simulink model "comunicacionesTarea2"  (R2021a)
settings: Solver=VariableStepAuto  StartTime=0.0  StopTime=0.5  RelTol=1e-3
libraries: spsTriangleGeneratorLib x1
settings Model: Creator=jmata  LastModifiedBy=jmata

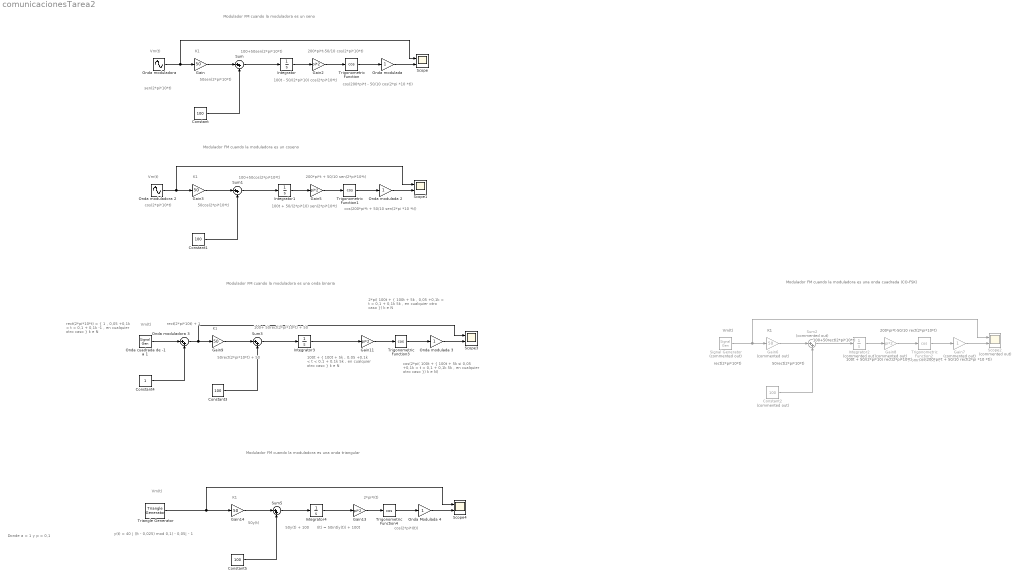
== system comunicacionesTarea2 ==
  note: cos(2*pi*I(t))
  note: 2*pi*I(t)
  note: I(t) = 50int(y(t)) + 100t
  note: 50y(t) + 100
  note: 50y(t)
  note: y(t) = 40 | ((t - 0,025) mod 0,1) - 0,05| - 1
  note: Donde a = 1 y p = 0,1
  note: 2*pi( 100t + {
      |
      | 100t + 5k , 0,05 +0,1k < t < 0,1 + 0,1k
      |
      | 5k , en cualquier otro caso
      |
      | }) k e N
  note: rect(2*pi*10t) + 1
  note: Modulador FM cuando la moduladora es una onda cuadrada (CO-FSK)
  note: Modulador FM cuando la moduladora es un coseno
  note: cos(200*pi*t - 50/10 cos(2*pi *10 *t))
  note: 200*pi*t-50/10 cos(2*pi*10*t)
  note: 100t - 50/(2*pi*10) cos(2*pi*10*t)
  note: 100+50sen(2*pi*10*t)
  note: 50sen(2*pi*10*t)
  note: sen(2*pi*10*t)
  note: Modulador FM cuando la moduladora es un seno
  note: K1
  note: Vm(t)
  note: 50cos(2*pi*10*t)
  note: 100t + 50/(2*pi*10) sen(2*pi*10*t)
  note: 100+50cos(2*pi*10*t)
  note: K1
  note: Vm(t)
  note: cos(200*pi*t + 50/10 sen(2*pi *10 *t))
  note: cos(2*pi*10*t)
  note: 200*pi*t + 50/10 sen(2*pi*10*t)
  note: 100+50rect(2*pi*10*t)
  note: rect(2*pi*10*t)
  note: cos(200*pi*t + 50/10 rect(2*pi *10 *t))
  note: 50rect(2*pi*10*t)
  note: 100t + 50/(2*pi*10) rect(2*pi*10*t)
  note: 200*pi*t-50/10 rect(2*pi*10*t)
  note: K1
  note: Vm(t)
  note: 50rect(2*pi*10*t) + 50
  note: 100+ 50rect(2*pi*10*t) + 50
  note: 100t + {
      |
      | 100t + 5k , 0,05 +0,1k < t < 0,1 + 0,1k
      |
      | 5k , en cualquier otro caso
      |
      | } k e N
  note: K1
  note: cos(2*pi( 100t + {
      |
      | 100t + 5k si 0,05 +0,1k < t < 0,1 + 0,1k
      |
      | 5k , en cualquier otro caso
      |
      | }) k e N)
  note: Vm(t)
  note: Modulador FM cuando la moduladora es una onda binaria
  note: K1
  note: Vm(t)
  note: Modulador FM cuando la moduladora es una onda triangular
  note: rect(2*pi*10*t) = {
      |
      | 1 , 0,05 +0,1k < t < 0,1 + 0,1k
      |
      | -1 , en cualquier otro caso
      |
      | } k e N
  Constant{,1,3,5} (4 alike) : Constant  Value=100
  Constant2 : Constant  Commented=on  Value=100
  Constant4 : Constant
  Gain{,3,9,14} (4 alike) : Gain  Gain=50
  Gain{2,5,11,13} (4 alike) : Gain  Gain=pi*2
  Gain6 : Gain  Commented=on  Gain=50
  Gain7 : Gain  Commented=on
  Gain8 : Gain  Commented=on  Gain=pi*2
  Integrator{,1,3..4} (4 alike) : Integrator
  Integrator2 : Integrator  Commented=on
  Onda Modulada 4 : Gain
  Onda cuadrada de -1 a 1 : SignalGenerator  WaveForm=square  Frequency=2*pi*10  Units=rad/sec
  Onda modulada : Gain
  Onda modulada 2 : Gain
  Onda modulada 3 : Gain
  Onda moduladora : Sin  Frequency=2*pi*10  SampleTime=1/10000
  Onda moduladora 2 : Sin  Frequency=2*pi*10  Phase=90  SampleTime=1/10000
  Onda moduladora 3 : Sum  Inputs=|++
  Scope{,1,3..4} (4 alike) : Scope  NumInputPorts=2
  Scope2 : Scope  Commented=on  NumInputPorts=2
  Signal Generator : SignalGenerator  Commented=on  WaveForm=square  Frequency=2*pi*10  Units=rad/sec
  Sum{,1,3,5} (4 alike) : Sum  Inputs=|++
  Sum2 : Sum  Commented=on  Inputs=|++
  Triangle Generator : spsTriangleGeneratorLib/Triangle Generator  Freq=10  Phase=0  Ts=0
  Trigonometric Function{,1,3..4} (4 alike) : Trigonometry  Operator=cos
  Trigonometric Function2 : Trigonometry  Commented=on  Operator=cos
  wires:
  Onda moduladora/1 -> Scope/1, Gain/1
  Constant/1 -> Sum/2
  Sum/1 -> Integrator/1
  Trigonometric Function/1 -> Onda modulada/1
  Onda modulada/1 -> Scope/2
  Integrator/1 -> Gain2/1
  Gain2/1 -> Trigonometric Function/1
  Gain/1 -> Sum/1
  Trigonometric Function1/1 -> Onda modulada 2/1
  Integrator1/1 -> Gain5/1
  Onda modulada 2/1 -> Scope1/2
  Gain3/1 -> Sum1/1
  Constant1/1 -> Sum1/2
  Sum1/1 -> Integrator1/1
  Gain5/1 -> Trigonometric Function1/1
  Onda moduladora 2/1 -> Scope1/1, Gain3/1
  Gain7/1 -> Scope2/2
  Sum2/1 -> Integrator2/1
  Signal Generator/1 -> Scope2/1, Gain6/1
  Gain8/1 -> Trigonometric Function2/1
  Gain6/1 -> Sum2/1
  Constant2/1 -> Sum2/2
  Integrator2/1 -> Gain8/1
  Trigonometric Function2/1 -> Gain7/1
  Gain11/1 -> Trigonometric Function3/1
  Onda modulada 3/1 -> Scope3/2
  Trigonometric Function3/1 -> Onda modulada 3/1
  Constant3/1 -> Sum3/2
  Gain9/1 -> Sum3/1
  Integrator3/1 -> Gain11/1
  Sum3/1 -> Integrator3/1
  Onda cuadrada de -1 a 1/1 -> Onda moduladora 3/1
  Constant4/1 -> Onda moduladora 3/2
  Onda moduladora 3/1 -> Scope3/1, Gain9/1
  Sum5/1 -> Integrator4/1
  Integrator4/1 -> Gain13/1
  Gain14/1 -> Sum5/1
  Constant5/1 -> Sum5/2
  Trigonometric Function4/1 -> Onda Modulada 4/1
  Onda Modulada 4/1 -> Scope4/2
  Gain13/1 -> Trigonometric Function4/1
  Triangle Generator/1 -> Scope4/1, Gain14/1
